simulink model "narx"  (R2019a)
settings: Solver=VariableStepAuto  StartTime=0.0  StopTime=10.0  RelTol=1e-3
libraries: neural x208
(part 2 of 4)

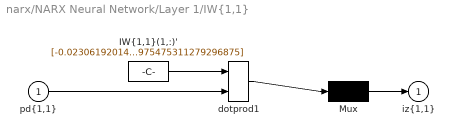
== system narx/NARX Neural Network/Layer 1/IW{1,1} ==
  "pd{1,1}" : Inport  PortDimensions=400  SampleTime=0.1
      mask Display: e = 0.06;c1 = [120 230 180]/255;c2 = ([120 230 180]+0)/(256+128);c3 = ([120 230 180]+128)/(256+128);patch([0 1 1 0],[0 0 1 1],c1);patch([0 1 1 1-e 1-e 0+e],[0 0 1 1-e 0+e 0+e],c2);patch([0 0 1 1-e 0+e 0+e],[0 1 1 1-e 1-e 0+e],c3);plot([0 1 1 0 0],[0 0 1 1 0]);
  "IW{1,1}(1,:)'" : Constant  Value=[-0.0230619201437031844104108557758081587962806224822998046875;-0.01203166708776239046674305654960335232317447662353515625;-0.01261812331188348623722816910230903886258602142333984375;-0.08363940243062374657601054650513106025755405426025390625;-0.03326307825413914176504448505511390976607799530029296875;-0.039726731679532938101839789624136756174266338348388671875;0.06382106758491161435653538092083181254565715789794921875;0.03794629846810058937389698030528961680829524993896484375;-0.0467220946135251669062427026801742613315582275390625;-0.0321588679729853665900662917920271866023540496826171875;0.083210834189238636060537146477145142853260040283203125;0.07671340216037876580390530989461694844067096710205078125;0.04748144901320051902704477697625407017767429351806640625;0.05756200100013088294392815669198171235620975494384765625;-0.076938512926083280074607273490983061492443084716796875;-0.0619295863528098455841330860494053922593593597412109375;0.00086531536179440776516968991671774347196333110332489013671875;0.03035442448645096769066498154643340967595577239990234375;-0.056106424472942569015021518907815334387123584747314453125;-0.01893134320386591351592642240575514733791351318359375;0.07271045420883136267686808196231140755116939544677734375;0.08031638656646129803551303893982549197971820831298828125;0.045234724325120316545945087227664771489799022674560546875;-0.073947112056574726413060716367908753454685211181640625;-0.0132330403076222034852715836450443021021783351898193359375;-0.05574608031008058961486284488273668102920055389404296875;-0.0415048058894514626526728306998847983777523040771484375;-0.01432425217057038679957514659690787084400653839111328125;-0.046261518060095686843968820767258876003324985504150390625;-0.056935736500312035535120713802825775928795337677001953125;-0.01121129358718043513010176326361033716239035129547119140625;-0.047574796371540044315207040881432476453483104705810546875;0.07772926784205387573667422884682309813797473907470703125;-0.0211245087994867686287392416488728486001491546630859375;-0.0242811741790668438045752708376312511973083019256591796875;0.08531958291325413001882083108284859918057918548583984375;-0.0300765308351161435307385971782423439435660839080810546875;0.068175559936289598095271458078059367835521697998046875;-0.022435939217997684369532152004467207007110118865966796875;-0.0861919205570601254517981715252972207963466644287109375;0.045383684360200272911445296131205395795404911041259765625;-0.01259936307395949361964682111647562123835086822509765625;-0.06402677338207841961637001304552541114389896392822265625;0.061179391862942945901071567504914128221571445465087890625;-0.004989141040821358334678148338525716098956763744354248046875;-0.084356312880124073583232302553369663655757904052734375;0.07627096263767001171895998368199798278510570526123046875;-0.021150871774745498565817314329251530580222606658935546875;0.06383078384680655747995814408568548969924449920654296875;0.06479993942444185750506591148223378695547580718994140625;-0.08285147770107560705188376459773280657827854156494140625;0.0649816211890949790852545220332103781402111053466796875;0.06435578507044560636618513171924860216677188873291015625;-0.0680156816615344050891422966742538847029209136962890625;0.079781954481924544086979267376591451466083526611328125;-0.0146783156336936539132498324988773674704134464263916015625;0.07248252569425893410137717864927253685891628265380859375;0.00632893548050383371317284542101333499886095523834228515625;-0.043498065872452383595625491352620883844792842864990234375;0.049019816202009382222204436629908741451799869537353515625;0.0176209883730439088866948083023089566268026828765869140625;-0.05128642132312975776553543028057902120053768157958984375;-0.021337479507201571882202273400253034196794033050537109375;-0.07527082428609037367817080621534842066466808319091796875;0.08468124030384889533440428976973635144531726837158203125;0.00295439731888423422201395140973545494489371776580810546875 ...(+20031 chars)]
      mask Display: e = 0.06;c1 = [120 150 230]/255;c2 = ([120 150 230]+0)/383;c3 = ([120 150 230]+128)/383;patch([0 1 1 0],[0 0 1 1],c1);patch([0 1 1 1-e 1-e 0+e],[0 0 1 1-e 0+e 0+e],c2);patch([0 0 1 1-e 0+e 0+e],[0 1 1 1-e 1-e 0+e],c3);plot([0 1 1 0 0],[0 0 1 1 0]);disp('Weights');
  Mux : Mux  Inputs=1
      mask Display: e = 0.06;c1 = [120 150 230]/255;c2 = ([120 150 230]+0)/383;c3 = ([120 150 230]+128)/383;patch([0 1 1 0],[0 0 1 1],c1);patch([0 1 1 1-e 1-e 0+e],[0 0 1 1-e 0+e 0+e],c2);patch([0 0 1 1-e 0+e 0+e],[0 1 1 1-e 1-e 0+e],c3);plot([0 1 1 0 0],[0 0 1 1 0]);disp('Mux');
  dotprod1 : neural/Weight Functions/dotprod
      settings: SourceProductName=MATLAB Runtime - Deep Learning Toolbox  SourceProductBaseCode=Missing
  "iz{1,1}" : Outport
      mask Display: e = 0.06;c1 = [120 230 180]/255;c2 = ([120 230 180]+0)/(256+128);c3 = ([120 230 180]+128)/(256+128);patch([0 1 1 0],[0 0 1 1],c1);patch([0 1 1 1-e 1-e 0+e],[0 0 1 1-e 0+e 0+e],c2);patch([0 0 1 1-e 0+e 0+e],[0 1 1 1-e 1-e 0+e],c3);plot([0 1 1 0 0],[0 0 1 1 0]);
  wires:
  "IW{1,1}(1,:)'"/1 -> dotprod1/1
  "pd{1,1}"/1 -> dotprod1/2
  dotprod1/1 -> Mux/1
  Mux/1 -> "iz{1,1}"/1
